simulink model "LLC"  (R2022b)
settings: Solver=VariableStepAuto  StartTime=0.0  StopTime=10.0  RelTol=1e-3
settings Model: Creator=Mohammad Khaled  LastModifiedBy=Mohammad Khaled

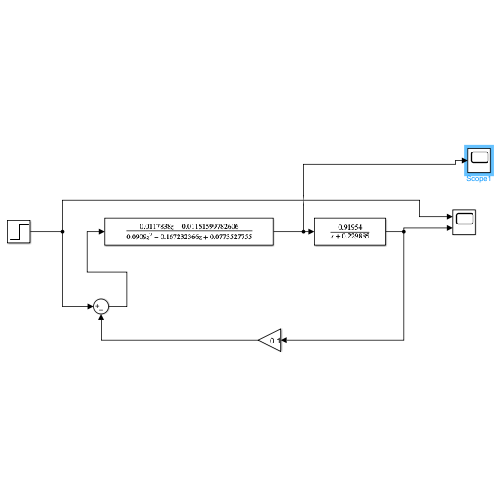
[thumbnail: Simulink's stored preview of the top-level diagram]
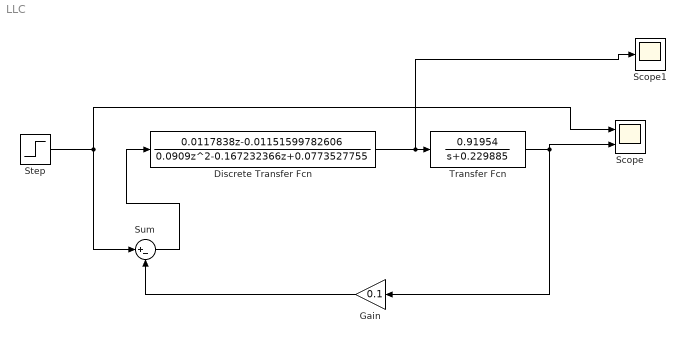
== system LLC ==
  Discrete Transfer Fcn : DiscreteTransferFcn  Numerator=[0.0117838 -0.01151599782606]  Denominator=[0.0909 -0.167232366 0.0773527755]  SampleTime=0.1
  Gain : Gain  Gain=0.1
  Scope : Scope  NumInputPorts=2
  Scope1 : Scope
  Step : Step  After=50  SampleTime=0
  Sum : Sum  Inputs=|+-
  Transfer Fcn : TransferFcn  Numerator=[0.91954]  Denominator=[1 0.229885]
  wires:
  Transfer Fcn/1 -> Scope/2, Gain/1
  Discrete Transfer Fcn/1 -> Scope1/1, Transfer Fcn/1
  Gain/1 -> Sum/2
  Step/1 -> Scope/1, Sum/1
  Sum/1 -> Discrete Transfer Fcn/1
